simulink model "FinalProjectModel"  (R2024a)
settings: Solver=ode1  StartTime=0.0  StopTime=Inf  FixedStep=1  RelTol=1e-3
PostLoadFcn:
  | , if any(exist('dsrtsu_mdlpostloadfcn', 'file') == [2, 3, 6]), try dsrtsu_mdlpostloadfcn('Execute', bdroot); catch fprintf('Error in PostLoadFcn (dsrtsu_mdlpostloadfcn) for model "%s":\n %s\n', bdroot, lasterr); end, end,
StartFcn:
  | %The GUI handles are by default hidden, turn them on
  | set(0,'ShowHiddenHandles','on');
  | 
  | %Set up the arguments that will go into the gain block event callback listener
  | blk = 'FinalProjectModel/Gain';
  | event = 'PostOutputs';
  | listener = @updategui;
  | 
  | %Create the listener
  | h = add_exec_event_listener(blk, event, listener);
values from neighbouring files (symbols this model uses):
  AuthKeyInput = str2num(get(handles.AuthKey,'String'))    [GUI_4SimulinkModel.m]
  ObjectDetectionInput = str2num(get(handles.ObjectDetection,'String'))    [GUI_4SimulinkModel.m]
undefined symbols (not defined in the file or in its folder): AccelPdlInput, BrkPdlInput, DistanceFromObject
libraries: simulink x4
Description:
  | Standard RTI1006 template.
  | Supported Matlab version:  R2017a.
settings Model: Tag=RTI1006  DSRTSU_INTERNAL_RTI_VER=500  DSRTSU_INTERNAL_RTI_TYPE=rti1006  RTICANMMDATA=struct('GeneralSetupData',struct('modelroot',['C:\Users\HZ8DGH\Documents\umich\Intelligent Vehicle Systems\FinalProject'],'generalsettings',struct('filesettings',struct('destfolder',struct('Name','RTICANMM_FILES','Check',1),'buildfolder',struct('Name','.','Check',1),'AbsDestfolder',struct('Name',['C:\Users\HZ8DGH\Documents\umich\Intelligent Vehicle Systems\FinalProject\RTICANMM_FILES']),'AbsBuildfolder',struct('Name',['C:\Users\HZ8DGH\Documents\umich\Intelligent Vehicle Systems\FinalProject']))),'options',struct('addpaths',1,'rmpaths',1,'addtrcexclusion',logical(1),'cannavigator',struct('checkmonitoring',0),'show_usrtrc',0,'use_usrtrc',0),'advanced',struct('options',ones(1,100)),'MPSetup',{{}},'modelname','vehicleModel','block','vehicleModel'))  DSRTSU_INTERNAL_RTIFLEXRAYCONFIG=110  DSRTSU_INTERNAL_RTIFPGA=90  Creator=HZ8DGH  LastModifiedBy=shaur
settings SolverCC: AlgebraicLoopSolver=TrustRegion
settings DataIOCC: ReturnWorkspaceOutputs=off
settings OptimizationCC: BlockReduction=off  OptimizeBlockIOStorage=off  BufferReuse=off  GlobalBufferReuse=off  ExpressionFolding=off  LocalBlockOutputs=off
settings DebuggingCC: UnconnectedInputMsg=warning  UnconnectedOutputMsg=warning  UnconnectedLineMsg=warning  ArithmeticOperatorsInVariantConditions=warning
settings HardwareCC: ProdBitPerPointer=32  ProdBitPerSizeT=32  ProdBitPerPtrDiffT=32  ProdLargestAtomicInteger=Integer  ProdWordSize=32  ProdHWDeviceType=Custom Processor->Custom  TargetIntDivRoundTo=Zero  TargetEndianess=LittleEndian  TargetHWDeviceType=Custom Processor->Custom
settings ModelReferenceCC: EnableRefExpFcnMdlSchedulingChecks=on
settings SFSimCC: SimUseLocalCustomCode=off  MATLABDynamicMemAlloc=off  CustomCodeUndefinedFunction=UseInterfaceOnly
settings RTWCC: Description=dSPACE DS1006 Hardware Platform  SystemTargetFile=rti1006.tlc  MakeCommand=make_rti  TemplateMakefile=rti1006.tmf  RTWUseLocalCustomCode=off  GPUComputeCapability=3.5
settings CodeAppCC: StateflowObjectComments=on
settings STFCustomTargetCC: TargetLangStandard=C89/C90 (ANSI)  ParMdlRefBuildCompliant=on  MatFileLogging=on  GRTInterface=off  UseToolchainInfoCompliant=off  SystemTargetFile=rti1006.tlc
settings GRTTargetCC: TargetLangStandard=C89/C90 (ANSI)  CompOptLevelCompliant=off  ConcurrentExecutionCompliant=off  CombineOutputUpdateFcns=off  CPPClassGenCompliant=off  UseToolchainInfoCompliant=off
settings ConfigComp: CovMetricSettings=dswe
settings SimscapeCC: SimscapeNormalizeSystem=off

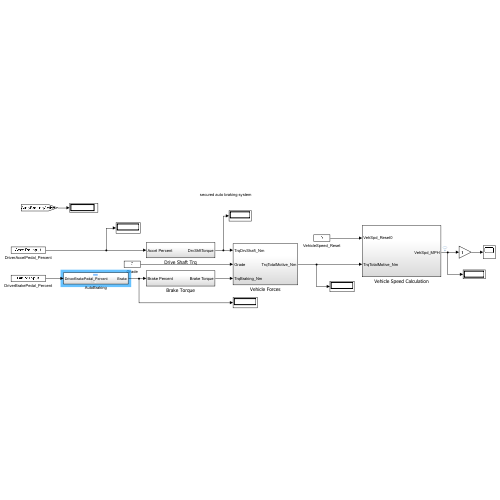
[thumbnail: Simulink's stored preview of the top-level diagram]
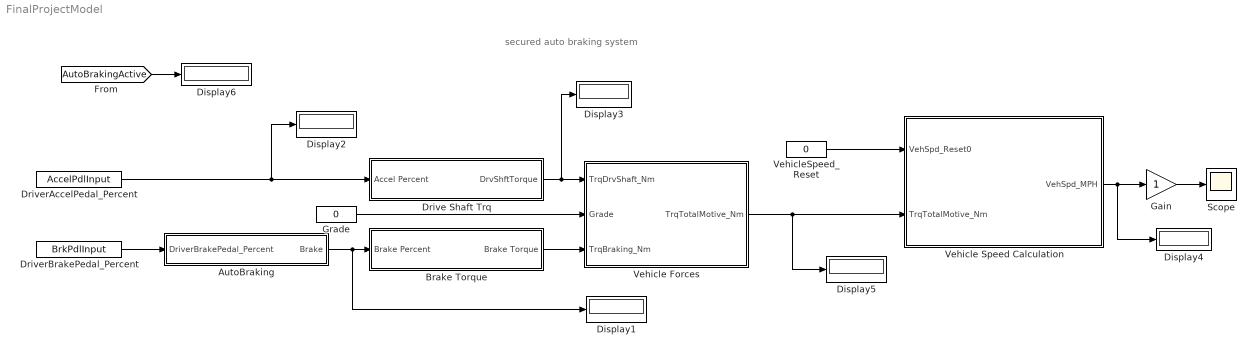
== system FinalProjectModel ==
  note: secured auto braking system
  AutoBraking : Subsystem
  Brake Torque : Subsystem
  Display{1..6} (6 alike) : Display
  Drive Shaft Trq : Subsystem
  DriverAccelPedal_Percent : Constant  Value=AccelPdlInput
  DriverBrakePedal_Percent : Constant  Value=BrkPdlInput
  Gain : Gain
  Grade : Constant  Value=0
  Scope : Scope
  Vehicle Forces : Subsystem
  Vehicle Speed Calculation : Subsystem
  VehicleSpeed_Reset : Constant  Value=0
  wires:
  DriverBrakePedal_Percent/1 -> AutoBraking/1(DriverBrakePedal_Percent)
  Vehicle Forces/1(TrqTotalMotive_Nm) -> Display5/1, Vehicle Speed Calculation/2(TrqTotalMotive_Nm)
  DriverAccelPedal_Percent/1 -> Display2/1, Drive Shaft Trq/1(Accel Percent)
  Grade/1 -> Vehicle Forces/2(Grade)
  VehicleSpeed_Reset/1 -> Vehicle Speed Calculation/1(VehSpd_Reset0)
  Brake Torque/1(Brake Torque) -> Vehicle Forces/3(TrqBraking_Nm)
  Drive Shaft Trq/1(DrvShftTorque) -> Display3/1, Vehicle Forces/1(TrqDrvShaft_Nm)
  Vehicle Speed Calculation/1(VehSpd_MPH) -> Display4/1, Gain/1
  AutoBraking/1(Brake) -> Display1/1, Brake Torque/1(Brake Percent)
  Gain/1 -> Scope/1
  [AutoBrakingActive] -> Display6/1

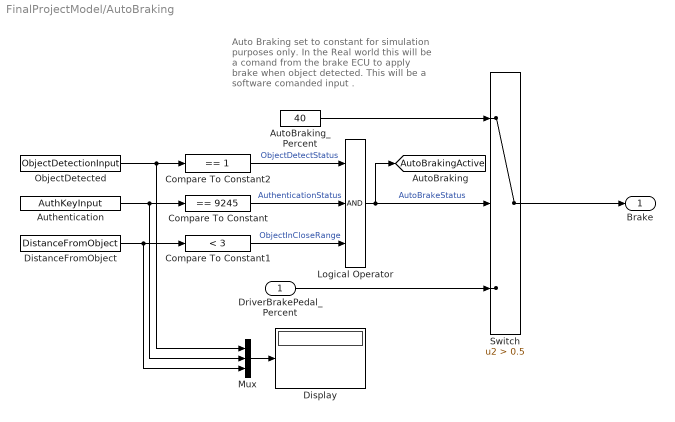
== system FinalProjectModel/AutoBraking ==
  note: Auto Braking set to constant for simulation purposes only. In the Real world this will be a comand from the brake ECU to apply brake when object detected. This will be a software comanded input
      |
      | .
  DriverBrakePedal_Percent : Inport
  Authentication : Constant  Value=AuthKeyInput
  AutoBraking_Percent : Constant  Value=40
  Compare To Constant : simulink/Logic and Bit Operations/Compare To Constant  relop===  const=9245  OutDataTypeStr=boolean
  Compare To Constant1 : simulink/Logic and Bit Operations/Compare To Constant  relop=<  const=3  OutDataTypeStr=boolean
  Compare To Constant2 : simulink/Logic and Bit Operations/Compare To Constant  relop===  const=1  OutDataTypeStr=boolean
  Display : Display
  DistanceFromObject : Constant  Value=DistanceFromObject
  Logical Operator : Logic  Inputs=3  AllPortsSameDT=off  OutDataTypeStr=boolean
  Mux : Mux  Inputs=3
  ObjectDetected : Constant  Value=ObjectDetectionInput
  Switch : Switch  Criteria=u2 > Threshold  Threshold=0.5  SaturateOnIntegerOverflow=off  InputSameDT=off
  Brake : Outport
  tag scope: AutoBrakingActive=global
  wires:
  DriverBrakePedal_Percent/1 -> Switch/3
  ObjectDetected/1 -> Compare To Constant2/1, Mux/1
  AutoBraking_Percent/1 -> Switch/1
  Logical Operator/1 -> [AutoBrakingActive], Switch/2  "AutoBrakeStatus"
  Authentication/1 -> Compare To Constant/1, Mux/2
  Compare To Constant/1 -> Logical Operator/2  "AuthenticationStatus"
  Switch/1 -> Brake/1
  DistanceFromObject/1 -> Compare To Constant1/1, Mux/3
  Compare To Constant1/1 -> Logical Operator/3  "ObjectInCloseRange"
  Mux/1 -> Display/1
  Compare To Constant2/1 -> Logical Operator/1  "ObjectDetectStatus"

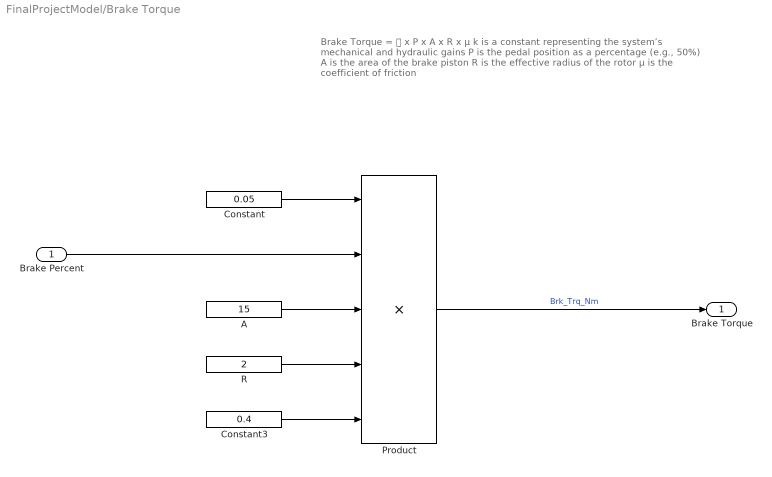
== system FinalProjectModel/Brake Torque ==
  note: Brake Torque = 𝑘 x P x A x R x μ
      |
      | k is a constant representing the system’s mechanical and hydraulic gains
      | P is the pedal position as a percentage (e.g., 50%)
      | A is the area of the brake piston
      | R is the effective radius of the rotor
      | μ is the coefficient of friction
  Brake Percent : Inport
  A : Constant  Value=15
  Constant : Constant  Value=0.05
  Constant3 : Constant  Value=0.4
  Product : Product  Inputs=5
  R : Constant  Value=2
  Brake Torque : Outport
  wires:
  Brake Percent/1 -> Product/2
  Constant/1 -> Product/1
  A/1 -> Product/3
  R/1 -> Product/4
  Constant3/1 -> Product/5
  Product/1 -> Brake Torque/1  "Brk_Trq_Nm"

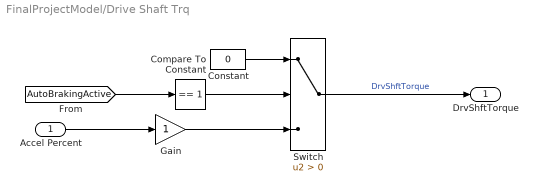
== system FinalProjectModel/Drive Shaft Trq ==
  Accel Percent : Inport
  Compare To Constant : simulink/Logic and Bit Operations/Compare To Constant  relop===  const=1  OutDataTypeStr=boolean
  Constant : Constant  Value=0
  Gain : Gain
  Switch : Switch  Criteria=u2 > Threshold  SaturateOnIntegerOverflow=off  InputSameDT=off
  DrvShftTorque : Outport
  wires:
  Accel Percent/1 -> Gain/1
  Gain/1 -> Switch/3
  Compare To Constant/1 -> Switch/2
  [AutoBrakingActive] -> Compare To Constant/1
  Switch/1 -> DrvShftTorque/1  "DrvShftTorque"
  Constant/1 -> Switch/1

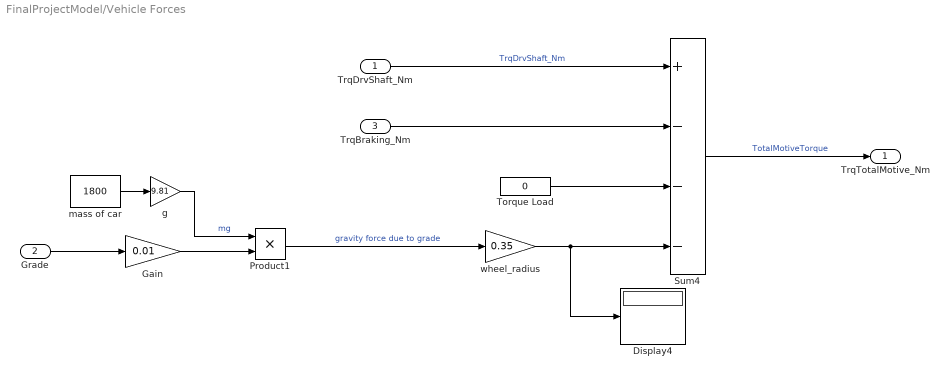
== system FinalProjectModel/Vehicle Forces ==
  TrqDrvShaft_Nm : Inport
  Grade : Inport  Port=2
  TrqBraking_Nm : Inport  Port=3
  Display4 : Display
  Gain : Gain  Gain=0.01  SaturateOnIntegerOverflow=on  OutDataTypeStr=Inherit: Same as input  ParamDataTypeStr=Inherit: Same as input
  Product1 : Product  InputSameDT=on  SaturateOnIntegerOverflow=on  OutDataTypeStr=Inherit: Same as first input
  Sum4 : Sum  Inputs=+---  InputSameDT=on  SaturateOnIntegerOverflow=on  OutDataTypeStr=Inherit: Same as first input
  Torque Load : Constant  Value=0
  g : Gain  Gain=9.81  SaturateOnIntegerOverflow=on  OutDataTypeStr=Inherit: Same as input  ParamDataTypeStr=Inherit: Same as input
  mass of car : Constant  Value=1800
  wheel_radius : Gain  Gain=0.35  SaturateOnIntegerOverflow=on  OutDataTypeStr=Inherit: Same as input  ParamDataTypeStr=Inherit: Same as input
  TrqTotalMotive_Nm : Outport
  wires:
  TrqBraking_Nm/1 -> Sum4/2
  Torque Load/1 -> Sum4/3
  TrqDrvShaft_Nm/1 -> Sum4/1  "TrqDrvShaft_Nm"
  wheel_radius/1 -> Display4/1, Sum4/4
  Sum4/1 -> TrqTotalMotive_Nm/1  "TotalMotiveTorque"
  Product1/1 -> wheel_radius/1  "gravity force due to grade"
  g/1 -> Product1/1  "mg"
  mass of car/1 -> g/1
  Gain/1 -> Product1/2
  Grade/1 -> Gain/1

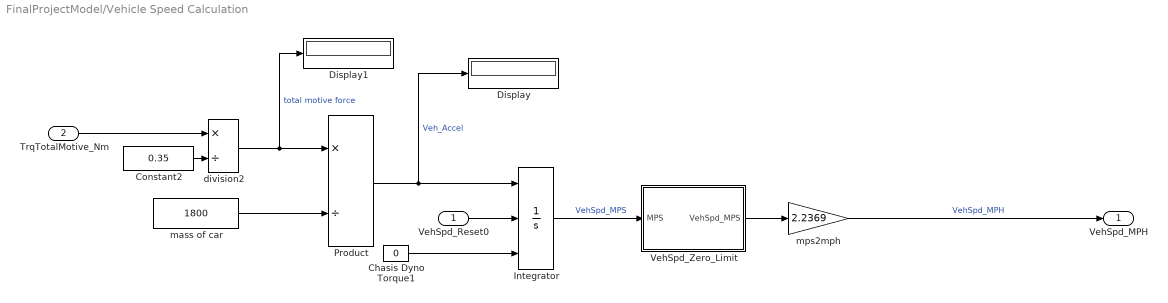
== system FinalProjectModel/Vehicle Speed Calculation ==
  VehSpd_Reset0 : Inport  OutDataTypeStr=double  PortDimensions=1
  TrqTotalMotive_Nm : Inport  Port=2
  Chasis Dyno Torque1 : Constant  Value=0
  Constant2 : Constant  Value=0.35
  Display : Display
  Display1 : Display
  Integrator : Integrator  ExternalReset=level hold  InitialConditionSource=external  LimitOutput=on  UpperSaturationLimit=100  LowerSaturationLimit=0
  Product : Product  Inputs=*/  InputSameDT=on  SaturateOnIntegerOverflow=on  OutDataTypeStr=Inherit: Same as first input
  VehSpd_Zero_Limit : Subsystem
  division2 : Product  Inputs=*/  InputSameDT=on  SaturateOnIntegerOverflow=on  OutDataTypeStr=Inherit: Same as first input
  mass of car : Constant  Value=1800
  mps2mph : Gain  Gain=2.2369  SaturateOnIntegerOverflow=on  OutDataTypeStr=Inherit: Same as input  ParamDataTypeStr=Inherit: Same as input
  VehSpd_MPH : Outport
  wires:
  VehSpd_Zero_Limit/1(VehSpd_MPS) -> mps2mph/1
  division2/1 -> Display1/1, Product/1  "total motive force"
  TrqTotalMotive_Nm/1 -> division2/1
  Constant2/1 -> division2/2
  mps2mph/1 -> VehSpd_MPH/1  "VehSpd_MPH"
  Integrator/1 -> VehSpd_Zero_Limit/1(MPS)  "VehSpd_MPS"
  Product/1 -> Display/1, Integrator/1  "Veh_Accel"
  mass of car/1 -> Product/2
  Chasis Dyno Torque1/1 -> Integrator/3
  VehSpd_Reset0/1 -> Integrator/2

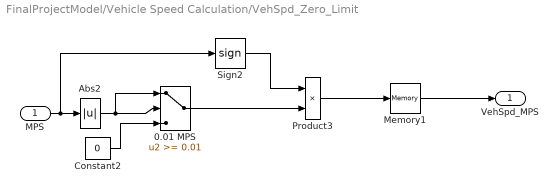
== system FinalProjectModel/Vehicle Speed Calculation/VehSpd_Zero_Limit ==
  MPS : Inport
  0.01 MPS : Switch  Threshold=0.01  SaturateOnIntegerOverflow=off  InputSameDT=off
  Abs2 : Abs
  Constant2 : Constant  Value=0
  Memory1 : Memory
  Product3 : Product  Inputs=**  InputSameDT=on  SaturateOnIntegerOverflow=on  OutDataTypeStr=Inherit: Same as first input
  Sign2 : Signum
  VehSpd_MPS : Outport
  wires:
  Memory1/1 -> VehSpd_MPS/1
  Product3/1 -> Memory1/1
  MPS/1 -> Abs2/1, Sign2/1
  Abs2/1 -> 0.01 MPS/2, 0.01 MPS/1
  Constant2/1 -> 0.01 MPS/3
  Sign2/1 -> Product3/1
  0.01 MPS/1 -> Product3/2
